simulink model "Model_2Systems"  (R2018b)
settings: Solver=ode23tb  StartTime=0.0  StopTime=20  RelTol=1e-3
values from neighbouring files (symbols this model uses):
  Ts = 0.01; Simulation.Ts = Ts    [Parameters.m]
undefined symbols (not defined in the file or in its folder): DiscIntNeverNeededParam, Kv, p01, p02, q01, q02, Simulation, Vr0
libraries: simulink x6
settings Model: Creator=oscar  LastModifiedBy=oscar
settings SolverCC: ZeroCrossAlgorithm=Adaptive
settings DataIOCC: OutputOption=SpecifiedOutputTimes  OutputTimes=t_out
settings SFSimCC: SimUseLocalCustomCode=off
settings RTWCC: RTWUseLocalCustomCode=off

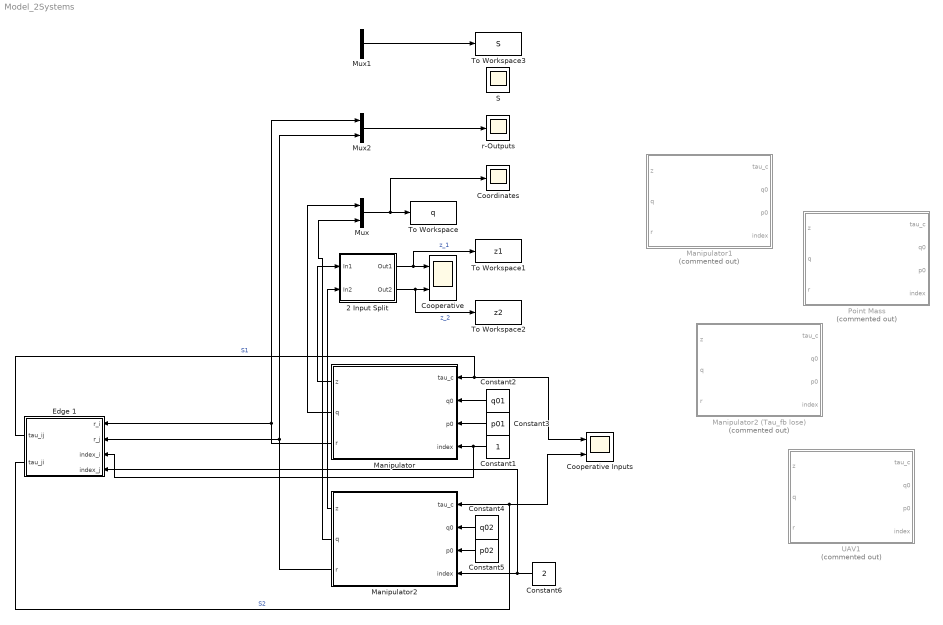
== system Model_2Systems ==
  2 Input Split : Subsystem
  Constant1 : Constant
  Constant2 : Constant  Value=q01
  Constant3 : Constant  Value=p01
  Constant4 : Constant  Value=q02
  Constant5 : Constant  Value=p02
  Constant6 : Constant  Value=2
  Cooperative : Scope  NumInputPorts=2
  Cooperative Inputs : Scope  NumInputPorts=2
  Coordinates : Scope
  Edge 1 : Subsystem
  Manipulator : Subsystem
  Manipulator1 : Subsystem  Commented=on
  Manipulator2 : Subsystem
  Manipulator2 (Tau_fb lose) : Subsystem  Commented=on
  Mux : Mux  Inputs=2
  Mux1 : Mux  Inputs=2
  Mux2 : Mux  Inputs=2
  Point Mass : Subsystem  Commented=on
  S : Scope  NumInputPorts=2
  To Workspace : ToWorkspace  VariableName=q  SaveFormat=Timeseries  SampleTime=-1
  To Workspace1 : ToWorkspace  VariableName=z1  SaveFormat=Timeseries  SampleTime=-1
  To Workspace2 : ToWorkspace  VariableName=z2  SaveFormat=Timeseries  SampleTime=-1
  To Workspace3 : ToWorkspace  VariableName=S  SaveFormat=Timeseries  SampleTime=-1
  UAV1 : Subsystem  Commented=on
  r-Outputs : Scope
  wires:
  Mux/1 -> Coordinates/1, To Workspace/1
  Manipulator/2(q) -> Mux/1
  Manipulator2/2(q) -> Mux/2
  Constant2/1 -> Manipulator/2(q0)
  Constant3/1 -> Manipulator/3(p0)
  Constant4/1 -> Manipulator2/2(q0)
  Constant5/1 -> Manipulator2/3(p0)
  Edge 1/1(tau_ij) -> Manipulator/1(tau_c), Cooperative Inputs/1  "S1"
  Edge 1/2(tau_ji) -> Manipulator2/1(tau_c), Cooperative Inputs/2  "S2"
  Manipulator2/3(r) -> Edge 1/2(r_j), Mux2/2
  Constant1/1 -> Manipulator/4(index), Edge 1/3(index_i)
  Constant6/1 -> Manipulator2/4(index), Edge 1/4(index_j)
  Manipulator/3(r) -> Edge 1/1(r_i), Mux2/1
  Mux2/1 -> r-Outputs/1
  Manipulator/1(z) -> 2 Input Split/1(In1)
  Manipulator2/1(z) -> 2 Input Split/2(In2)
  2 Input Split/1(Out1) -> To Workspace1/1, Cooperative/1  "z_1"
  2 Input Split/2(Out2) -> To Workspace2/1, Cooperative/2  "z_2"
  Mux1/1 -> To Workspace3/1

== system Model_2Systems/2 Input Split ==
  In1 : Inport
  In2 : Inport  Port=2
  Demux : Demux  Outputs=2
  Demux1 : Demux  Outputs=2
  Mux1 : Mux  Inputs=2
  Mux3 : Mux  Inputs=2
  Out1 : Outport
  Out2 : Outport  Port=2
  wires:
  Demux/1 -> Mux1/1
  Mux1/1 -> Out1/1
  In1/1 -> Demux/1
  Demux1/2 -> Mux3/2
  Mux3/1 -> Out2/1
  Demux1/1 -> Mux1/2
  Demux/2 -> Mux3/1
  In2/1 -> Demux1/1

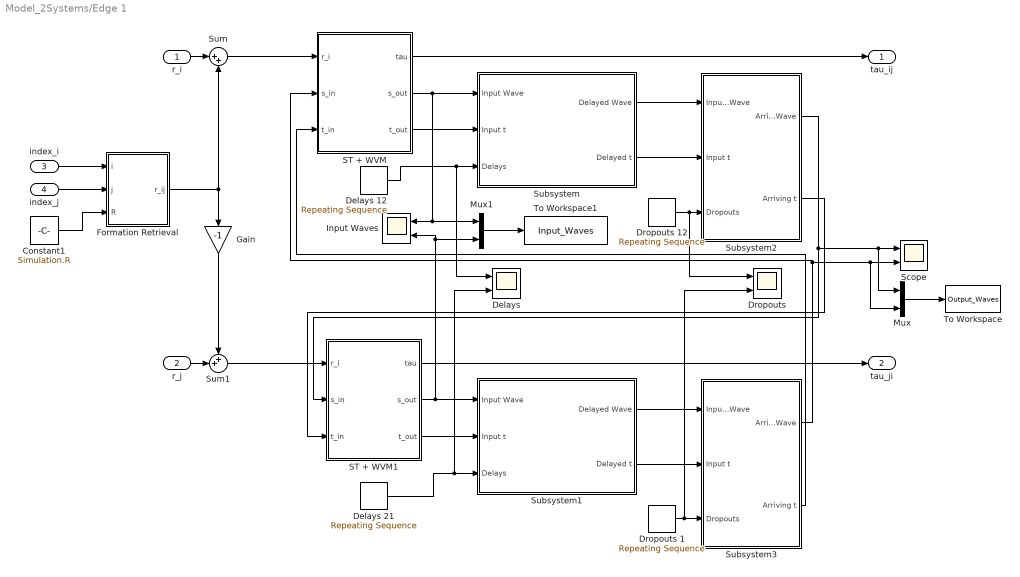
== system Model_2Systems/Edge 1 ==
  r_i : Inport
  r_j : Inport  Port=2
  index_i : Inport  Port=3
  index_j : Inport  Port=4
  Constant1 : Constant  Value=Simulation.R
  Delays : Scope  NumInputPorts=2
  Delays 12 : simulink/Sources/Repeating Sequence  rep_seq_t=t_delays  rep_seq_y=delays_12
  Delays 21 : simulink/Sources/Repeating Sequence  rep_seq_t=t_delays  rep_seq_y=delays_21
  Dropouts : Scope  NumInputPorts=2
  Dropouts 1 : simulink/Sources/Repeating Sequence  rep_seq_t=t_delays  rep_seq_y=dropouts_21
  Dropouts 12 : simulink/Sources/Repeating Sequence  rep_seq_t=t_delays  rep_seq_y=dropouts_12
  Formation Retrieval : MATLAB Function  TreatAsAtomicUnit=on
  Gain : Gain  Gain=-1
  Input Waves : Scope  NumInputPorts=2
  Mux : Mux  Inputs=2
  Mux1 : Mux  Inputs=2
  ST + WVM : Subsystem  TreatAsAtomicUnit=on
  ST + WVM1 : Subsystem  TreatAsAtomicUnit=on
  Scope : Scope  NumInputPorts=2
  Subsystem : Subsystem
  Subsystem1 : Subsystem
  Subsystem2 : Subsystem
  Subsystem3 : Subsystem
  Sum : Sum  Inputs=|++
  Sum1 : Sum  Inputs=++|
  To Workspace : ToWorkspace  VariableName=Output_Waves  SaveFormat=Timeseries  SampleTime=Ts
  To Workspace1 : ToWorkspace  VariableName=Input_Waves  SaveFormat=Timeseries  SampleTime=Ts
  tau_ij : Outport
  tau_ji : Outport  Port=2
  wires:
  r_i/1 -> Sum/1
  r_j/1 -> Sum1/2
  ST + WVM/1(tau) -> tau_ij/1
  Sum/1 -> ST + WVM/1(r_i)
  Sum1/1 -> ST + WVM1/1(r_i)
  index_i/1 -> Formation Retrieval/1(i)
  index_j/1 -> Formation Retrieval/2(j)
  Formation Retrieval/1(r_ij) -> Gain/1, Sum/2
  Gain/1 -> Sum1/1
  Constant1/1 -> Formation Retrieval/3(R)
  Delays 21/1 -> Delays/2, Subsystem1/3(Delays)
  ST + WVM/3(t_out) -> Subsystem/2(Input t)
  Delays 12/1 -> Delays/1, Subsystem/3(Delays)
  ST + WVM1/2(s_out) -> Subsystem1/1(Input Wave), Mux1/2, Input Waves/2
  ST + WVM1/3(t_out) -> Subsystem1/2(Input t)
  Subsystem/1(Delayed Wave) -> Subsystem2/1(Input Wave)
  ST + WVM1/1(tau) -> tau_ji/1
  Subsystem/2(Delayed t) -> Subsystem2/2(Input t)
  Dropouts 12/1 -> Dropouts/1, Subsystem2/3(Dropouts)
  Subsystem1/1(Delayed Wave) -> Subsystem3/1(Input Wave)
  Subsystem1/2(Delayed t) -> Subsystem3/2(Input t)
  Subsystem3/1(Arriving Wave) -> Mux/2, Scope/2, ST + WVM/2(s_in)
  Subsystem3/2(Arriving t) -> ST + WVM/3(t_in)
  Subsystem2/2(Arriving t) -> ST + WVM1/3(t_in)
  Subsystem2/1(Arriving Wave) -> ST + WVM1/2(s_in), Mux/1, Scope/1
  Dropouts 1/1 -> Subsystem3/3(Dropouts), Dropouts/2
  Mux/1 -> To Workspace/1
  ST + WVM/2(s_out) -> Subsystem/1(Input Wave), Input Waves/1, Mux1/1
  Mux1/1 -> To Workspace1/1

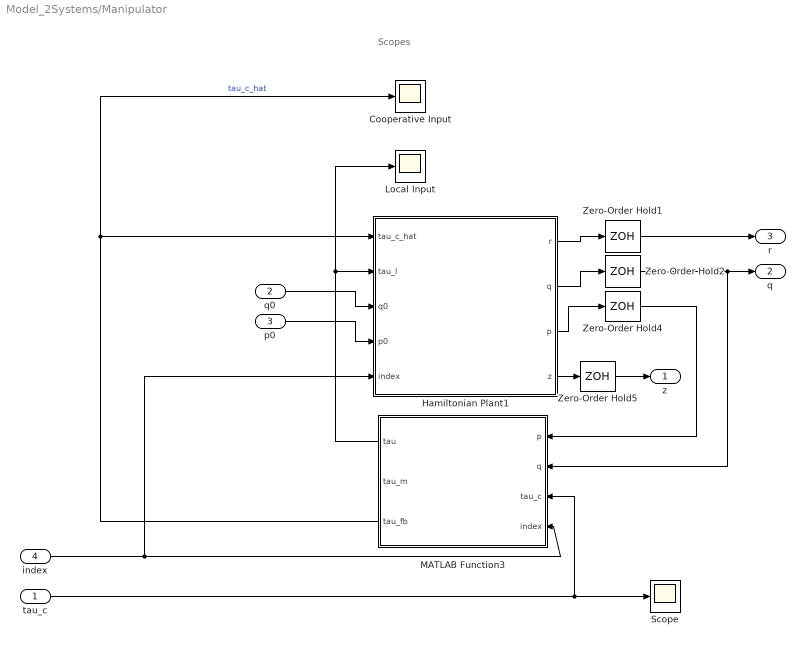
== system Model_2Systems/Manipulator ==
  note: Scopes
  tau_c : Inport
  q0 : Inport  Port=2
  p0 : Inport  Port=3
  index : Inport  Port=4
  Cooperative Input : Scope
  Hamiltonian Plant1 : Subsystem
  Local Input : Scope
  MATLAB Function3 : MATLAB Function  TreatAsAtomicUnit=on
  Scope : Scope
  Zero-Order Hold{1..2,4..5} (4 alike) : ZeroOrderHold  SampleTime=Ts
  z : Outport
  q : Outport  Port=2
  r : Outport  Port=3
  wires:
  Hamiltonian Plant1/2(q) -> Zero-Order Hold2/1
  index/1 -> Hamiltonian Plant1/5(index), MATLAB Function3/4(index)
  Hamiltonian Plant1/1(r) -> Zero-Order Hold1/1
  MATLAB Function3/1(tau) -> Local Input/1, Hamiltonian Plant1/2(tau_l)
  Hamiltonian Plant1/4(z) -> Zero-Order Hold5/1
  p0/1 -> Hamiltonian Plant1/4(p0)
  MATLAB Function3/3(tau_fb) -> Cooperative Input/1, Hamiltonian Plant1/1(tau_c_hat)  "tau_c_hat"
  Hamiltonian Plant1/3(p) -> Zero-Order Hold4/1
  q0/1 -> Hamiltonian Plant1/3(q0)
  Zero-Order Hold2/1 -> MATLAB Function3/2(q), q/1
  Zero-Order Hold4/1 -> MATLAB Function3/1(p)
  Zero-Order Hold1/1 -> r/1
  tau_c/1 -> Scope/1, MATLAB Function3/3(tau_c)
  Zero-Order Hold5/1 -> z/1

== system Model_2Systems/Manipulator1 ==
  tau_c : Inport
  q0 : Inport  Port=2
  p0 : Inport  Port=3
  index : Inport  Port=4
  Hamiltonian Plant : Subsystem
  Input Compensation : Scope  NumInputPorts=2
  Levenberg Compensation : MATLAB Function  Commented=on  TreatAsAtomicUnit=on
  Local Input : Scope
  MATLAB Function1 : MATLAB Function  TreatAsAtomicUnit=on
  Passivating Feedback : Scope
  Sum : Sum  Inputs=|++
  z : Outport
  q : Outport  Port=2
  r : Outport  Port=3
  wires:
  MATLAB Function1/1(tau) -> Hamiltonian Plant/3(tau_l), Local Input/1
  Hamiltonian Plant/4(p) -> MATLAB Function1/1(p)
  Hamiltonian Plant/3(q) -> q/1, MATLAB Function1/2(q)
  Hamiltonian Plant/5(z) -> z/1
  Hamiltonian Plant/2(r) -> r/1
  q0/1 -> Hamiltonian Plant/4(q0)
  p0/1 -> Hamiltonian Plant/5(p0)
  MATLAB Function1/2(tau_fb) -> Sum/2, Passivating Feedback/1
  index/1 -> Hamiltonian Plant/6(index), MATLAB Function1/3(index)
  Sum/1 -> Hamiltonian Plant/2(tau_c_hat), Input Compensation/2, Input Compensation/1  "tau_k"
  tau_c/1 -> Sum/1, Hamiltonian Plant/7(tau_c)  "tau_c_hat"

== system Model_2Systems/Manipulator2 ==
  note: Scopes
  tau_c : Inport
  q0 : Inport  Port=2
  p0 : Inport  Port=3
  index : Inport  Port=4
  Cooperative Input : Scope
  Hamiltonian Plant1 : Subsystem
  Local Input : Scope
  MATLAB Function3 : MATLAB Function  TreatAsAtomicUnit=on
  Scope : Scope
  Zero-Order Hold{1..2,4..5} (4 alike) : ZeroOrderHold  SampleTime=Ts
  z : Outport
  q : Outport  Port=2
  r : Outport  Port=3
  wires:
  Hamiltonian Plant1/2(q) -> Zero-Order Hold2/1
  index/1 -> Hamiltonian Plant1/5(index), MATLAB Function3/4(index)
  Hamiltonian Plant1/1(r) -> Zero-Order Hold1/1
  MATLAB Function3/1(tau) -> Local Input/1, Hamiltonian Plant1/2(tau_l)
  Hamiltonian Plant1/4(z) -> Zero-Order Hold5/1
  p0/1 -> Hamiltonian Plant1/4(p0)
  MATLAB Function3/3(tau_fb) -> Cooperative Input/1, Hamiltonian Plant1/1(tau_c_hat)  "tau_c_hat"
  Hamiltonian Plant1/3(p) -> Zero-Order Hold4/1
  q0/1 -> Hamiltonian Plant1/3(q0)
  Zero-Order Hold2/1 -> MATLAB Function3/2(q), q/1
  Zero-Order Hold4/1 -> MATLAB Function3/1(p)
  Zero-Order Hold1/1 -> r/1
  tau_c/1 -> Scope/1, MATLAB Function3/3(tau_c)
  Zero-Order Hold5/1 -> z/1

== system Model_2Systems/Manipulator2 (Tau_fb lose) ==
  tau_c : Inport
  q0 : Inport  Port=2
  p0 : Inport  Port=3
  index : Inport  Port=4
  Hamiltonian Plant : Subsystem
  Levenberg Compensation : MATLAB Function  Commented=on  TreatAsAtomicUnit=on
  Local Input : Scope
  MATLAB Function1 : MATLAB Function  TreatAsAtomicUnit=on
  MATLAB Function2 : MATLAB Function  Commented=on  TreatAsAtomicUnit=on
  Passivating Feedback : Scope
  Scope : Scope  NumInputPorts=4
  Sum : Sum  Inputs=|++
  System Input : Scope
  z : Outport
  q : Outport  Port=2
  r : Outport  Port=3
  wires:
  MATLAB Function1/1(tau) -> Hamiltonian Plant/2(tau_l), Local Input/1
  Hamiltonian Plant/3(p) -> MATLAB Function1/1(p)
  Hamiltonian Plant/2(q) -> MATLAB Function1/2(q), q/1
  Hamiltonian Plant/4(z) -> z/1
  Hamiltonian Plant/1(r) -> r/1
  q0/1 -> Hamiltonian Plant/3(q0)
  p0/1 -> Hamiltonian Plant/4(p0)
  MATLAB Function1/5(tau_fb) -> Scope/4, Sum/2, Passivating Feedback/1
  index/1 -> MATLAB Function1/3(index), Hamiltonian Plant/5(index)
  Sum/1 -> Hamiltonian Plant/1(tau_c_hat), System Input/1  "tau_k"
  tau_c/1 -> Sum/1, Hamiltonian Plant/6(tau_c)  "tau_c_hat"
  MATLAB Function1/2(tau_dH) -> Scope/1
  MATLAB Function1/3(tau_null) -> Scope/2
  MATLAB Function1/4(tau_lambda) -> Scope/3

== system Model_2Systems/Point Mass ==
  tau_c : Inport
  q0 : Inport  Port=2
  p0 : Inport  Port=3
  index : Inport  Port=4
  Hamiltonian Plant : Subsystem
  MATLAB Function1 : MATLAB Function  TreatAsAtomicUnit=on
  Scope : Scope
  Sum : Sum  Inputs=|++
  z : Outport
  q : Outport  Port=2
  r : Outport  Port=3
  wires:
  MATLAB Function1/1(tau) -> Hamiltonian Plant/2(tau_l)
  tau_c/1 -> Sum/1
  Hamiltonian Plant/3(p) -> MATLAB Function1/1(p)
  Hamiltonian Plant/2(q) -> MATLAB Function1/2(q), q/1
  Hamiltonian Plant/4(z) -> z/1
  Hamiltonian Plant/1(r) -> r/1
  q0/1 -> Hamiltonian Plant/3(q0)
  p0/1 -> Hamiltonian Plant/4(p0)
  MATLAB Function1/2(tau_fb) -> Scope/1, Sum/2
  Sum/1 -> Hamiltonian Plant/1(tau_c)
  index/1 -> Hamiltonian Plant/5(index), MATLAB Function1/3(index)

== system Model_2Systems/UAV1 ==
  tau_c : Inport
  q0 : Inport  Port=2
  p0 : Inport  Port=3
  index : Inport  Port=4
  Hamiltonian Plant : Subsystem
  Levenberg Compensation : MATLAB Function  Commented=on  TreatAsAtomicUnit=on
  Local Input : Scope
  MATLAB Function1 : MATLAB Function  TreatAsAtomicUnit=on
  Passivating Feedback : Scope
  Sum : Sum  Inputs=|++
  System Input : Scope
  z : Outport
  q : Outport  Port=2
  r : Outport  Port=3
  wires:
  MATLAB Function1/1(tau) -> Hamiltonian Plant/2(tau_l), Local Input/1
  Hamiltonian Plant/2(q) -> MATLAB Function1/2(q), q/1
  Hamiltonian Plant/4(z) -> z/1
  Hamiltonian Plant/1(r) -> r/1
  q0/1 -> Hamiltonian Plant/3(q0)
  p0/1 -> Hamiltonian Plant/4(p0)
  MATLAB Function1/2(tau_fb) -> Sum/2, Passivating Feedback/1
  index/1 -> MATLAB Function1/3(index), Hamiltonian Plant/5(index)
  Sum/1 -> System Input/1, Hamiltonian Plant/1(tau_c_hat)  "tau_c_hat"
  tau_c/1 -> Hamiltonian Plant/6(tau_c), Sum/1
  Hamiltonian Plant/3(p) -> MATLAB Function1/1(p)

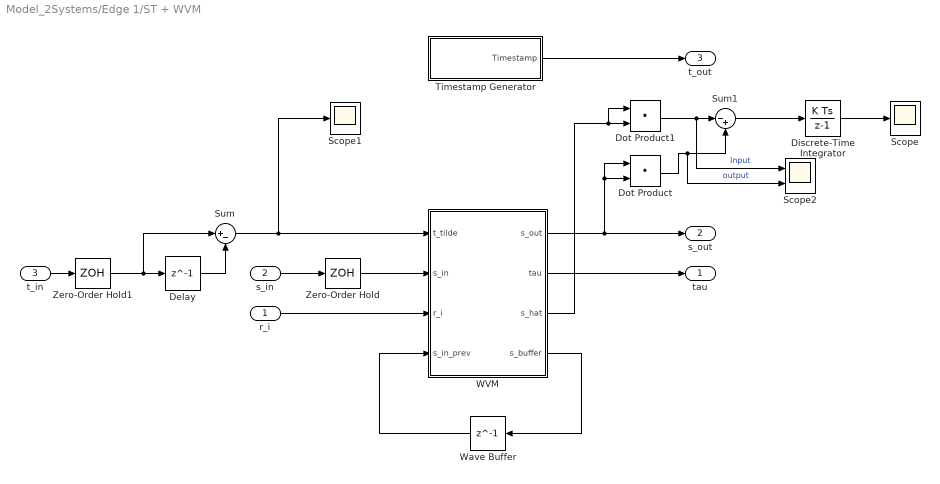
== system Model_2Systems/Edge 1/ST + WVM ==
  r_i : Inport
  s_in : Inport  Port=2
  t_in : Inport  Port=3
  Delay : Delay  DelayLength=1  SampleTime=Ts
  Discrete-Time Integrator : DiscreteIntegrator  SampleTime=-1  ICPrevOutput=DiscIntNeverNeededParam  ICPrevScaledInput=DiscIntNeverNeededParam
  Dot Product : DotProduct  InputSameDT=on  OutDataTypeStr=Inherit: Inherit via internal rule
  Dot Product1 : DotProduct  InputSameDT=on  OutDataTypeStr=Inherit: Inherit via internal rule
  Scope : Scope
  Scope1 : Scope
  Scope2 : Scope  NumInputPorts=2
  Sum : Sum  Inputs=|+-
  Sum1 : Sum  Inputs=|-+
  Timestamp Generator : Subsystem
  WVM : MATLAB Function  TreatAsAtomicUnit=on
  Wave Buffer : Delay  DelayLength=1  InitialCondition=[0;0]  SampleTime=Ts
  Zero-Order Hold : ZeroOrderHold  SampleTime=Ts
  Zero-Order Hold1 : ZeroOrderHold  SampleTime=Ts
  tau : Outport
  s_out : Outport  Port=2
  t_out : Outport  Port=3
  wires:
  t_in/1 -> Zero-Order Hold1/1
  Delay/1 -> Sum/2
  WVM/2(tau) -> tau/1
  WVM/1(s_out) -> Dot Product/2, Dot Product/1, s_out/1
  WVM/4(s_buffer) -> Wave Buffer/1
  Wave Buffer/1 -> WVM/4(s_in_prev)
  Sum/1 -> WVM/1(t_tilde), Scope1/1
  s_in/1 -> Zero-Order Hold/1
  r_i/1 -> WVM/3(r_i)
  WVM/3(s_hat) -> Dot Product1/1, Dot Product1/2
  Dot Product1/1 -> Scope2/1, Sum1/1  "Input"
  Dot Product/1 -> Scope2/2, Sum1/2  "output"
  Timestamp Generator/1(Timestamp) -> t_out/1
  Zero-Order Hold/1 -> WVM/2(s_in)
  Zero-Order Hold1/1 -> Sum/1, Delay/1
  Sum1/1 -> Discrete-Time Integrator/1
  Discrete-Time Integrator/1 -> Scope/1

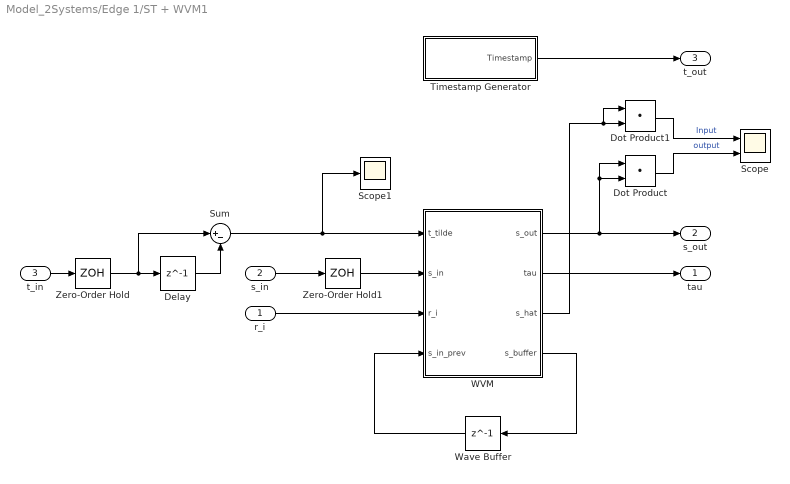
== system Model_2Systems/Edge 1/ST + WVM1 ==
  r_i : Inport
  s_in : Inport  Port=2
  t_in : Inport  Port=3
  Delay : Delay  DelayLength=1  SampleTime=Ts
  Dot Product : DotProduct  InputSameDT=on  OutDataTypeStr=Inherit: Inherit via internal rule
  Dot Product1 : DotProduct  InputSameDT=on  OutDataTypeStr=Inherit: Inherit via internal rule
  Scope : Scope  NumInputPorts=2
  Scope1 : Scope
  Sum : Sum  Inputs=|+-
  Timestamp Generator : Subsystem
  WVM : MATLAB Function  TreatAsAtomicUnit=on
  Wave Buffer : Delay  DelayLength=1  InitialCondition=[0;0]  SampleTime=Ts
  Zero-Order Hold : ZeroOrderHold  SampleTime=Ts
  Zero-Order Hold1 : ZeroOrderHold  SampleTime=Ts
  tau : Outport
  s_out : Outport  Port=2
  t_out : Outport  Port=3
  wires:
  t_in/1 -> Zero-Order Hold/1
  Delay/1 -> Sum/2
  WVM/2(tau) -> tau/1
  WVM/1(s_out) -> Dot Product/2, Dot Product/1, s_out/1
  WVM/4(s_buffer) -> Wave Buffer/1
  Wave Buffer/1 -> WVM/4(s_in_prev)
  Sum/1 -> Scope1/1, WVM/1(t_tilde)
  s_in/1 -> Zero-Order Hold1/1
  r_i/1 -> WVM/3(r_i)
  WVM/3(s_hat) -> Dot Product1/1, Dot Product1/2
  Dot Product1/1 -> Scope/1  "Input"
  Dot Product/1 -> Scope/2  "output"
  Timestamp Generator/1(Timestamp) -> t_out/1
  Zero-Order Hold1/1 -> WVM/2(s_in)
  Zero-Order Hold/1 -> Sum/1, Delay/1

== system Model_2Systems/Edge 1/Subsystem ==
  Input Wave : Inport
  Input t : Inport  Port=2
  Delays : Inport  Port=3
  Variable Integer Delay1 : Delay  DelayLengthSource=Input port  PreventDirectFeedthrough=on  SampleTime=Ts
      settings: InputPortMap=u0,p1
  Variable Integer Delay2 : Delay  DelayLengthSource=Input port  PreventDirectFeedthrough=on  SampleTime=Ts
      settings: InputPortMap=u0,p1
  Zero-Order Hold : ZeroOrderHold  SampleTime=Ts
  Delayed Wave : Outport
  Delayed t : Outport  Port=2
  wires:
  Input Wave/1 -> Variable Integer Delay2/1
  Input t/1 -> Variable Integer Delay1/1
  Variable Integer Delay2/1 -> Delayed Wave/1
  Variable Integer Delay1/1 -> Delayed t/1
  Delays/1 -> Zero-Order Hold/1
  Zero-Order Hold/1 -> Variable Integer Delay2/2, Variable Integer Delay1/2

== system Model_2Systems/Edge 1/Subsystem1 ==
  Input Wave : Inport
  Input t : Inport  Port=2
  Delays : Inport  Port=3
  Variable Integer Delay1 : Delay  DelayLengthSource=Input port  PreventDirectFeedthrough=on  SampleTime=Ts
      settings: InputPortMap=u0,p1
  Variable Integer Delay2 : Delay  DelayLengthSource=Input port  PreventDirectFeedthrough=on  SampleTime=Ts
      settings: InputPortMap=u0,p1
  Zero-Order Hold : ZeroOrderHold  SampleTime=Ts
  Delayed Wave : Outport
  Delayed t : Outport  Port=2
  wires:
  Input Wave/1 -> Variable Integer Delay2/1
  Zero-Order Hold/1 -> Variable Integer Delay2/2, Variable Integer Delay1/2
  Input t/1 -> Variable Integer Delay1/1
  Variable Integer Delay2/1 -> Delayed Wave/1
  Variable Integer Delay1/1 -> Delayed t/1
  Delays/1 -> Zero-Order Hold/1

== system Model_2Systems/Edge 1/Subsystem2 ==
  Input Wave : Inport
  Input t : Inport  Port=2
  Dropouts : Inport  Port=3
  Ground : Ground
  Ground1 : Ground
  Switch : Switch  Criteria=u2 > Threshold
  Switch1 : Switch  Criteria=u2 > Threshold
  Zero-Order Hold : ZeroOrderHold  SampleTime=Ts
  Arriving Wave : Outport
  Arriving t : Outport  Port=2
  wires:
  Input Wave/1 -> Switch/3
  Switch/1 -> Arriving Wave/1
  Switch1/1 -> Arriving t/1
  Dropouts/1 -> Zero-Order Hold/1
  Zero-Order Hold/1 -> Switch1/2, Switch/2
  Input t/1 -> Switch1/3
  Ground1/1 -> Switch/1
  Ground/1 -> Switch1/1

== system Model_2Systems/Edge 1/Subsystem3 ==
  Input Wave : Inport
  Input t : Inport  Port=2
  Dropouts : Inport  Port=3
  Ground1 : Ground
  Ground2 : Ground
  Switch : Switch  Criteria=u2 > Threshold
  Switch1 : Switch  Criteria=u2 > Threshold
  Zero-Order Hold : ZeroOrderHold  SampleTime=Ts
  Arriving Wave : Outport
  Arriving t : Outport  Port=2
  wires:
  Input Wave/1 -> Switch/3
  Switch/1 -> Arriving Wave/1
  Switch1/1 -> Arriving t/1
  Dropouts/1 -> Zero-Order Hold/1
  Zero-Order Hold/1 -> Switch1/2, Switch/2
  Input t/1 -> Switch1/3
  Ground1/1 -> Switch/1
  Ground2/1 -> Switch1/1

== system Model_2Systems/Manipulator/Hamiltonian Plant1 ==
  tau_c_hat : Inport
  tau_l : Inport  Port=2
  q0 : Inport  Port=3
  p0 : Inport  Port=4
  index : Inport  Port=5
  Integrator : Integrator  InitialConditionSource=external  InitialCondition=q01
  Integrator1 : Integrator  InitialConditionSource=external  InitialCondition=p02
  MATLAB Function1 : MATLAB Function  TreatAsAtomicUnit=on
  MATLAB Function2 : MATLAB Function  TreatAsAtomicUnit=on
  r : Outport
  q : Outport  Port=2
  p : Outport  Port=3
  z : Outport  Port=4
  wires:
  tau_l/1 -> MATLAB Function2/3(tau_l)
  MATLAB Function2/2(pdot) -> Integrator1/1
  Integrator1/1 -> MATLAB Function2/2(p), p/1, MATLAB Function1/2(p)
  Integrator/1 -> q/1, MATLAB Function2/1(q), MATLAB Function1/1(q)
  MATLAB Function2/1(qdot) -> Integrator/1
  p0/1 -> Integrator1/2
  q0/1 -> Integrator/2
  MATLAB Function1/1(z_out) -> z/1
  MATLAB Function1/2(r_out) -> r/1
  index/1 -> MATLAB Function1/3(index), MATLAB Function2/5(index)
  tau_c_hat/1 -> MATLAB Function2/4(tau_c)

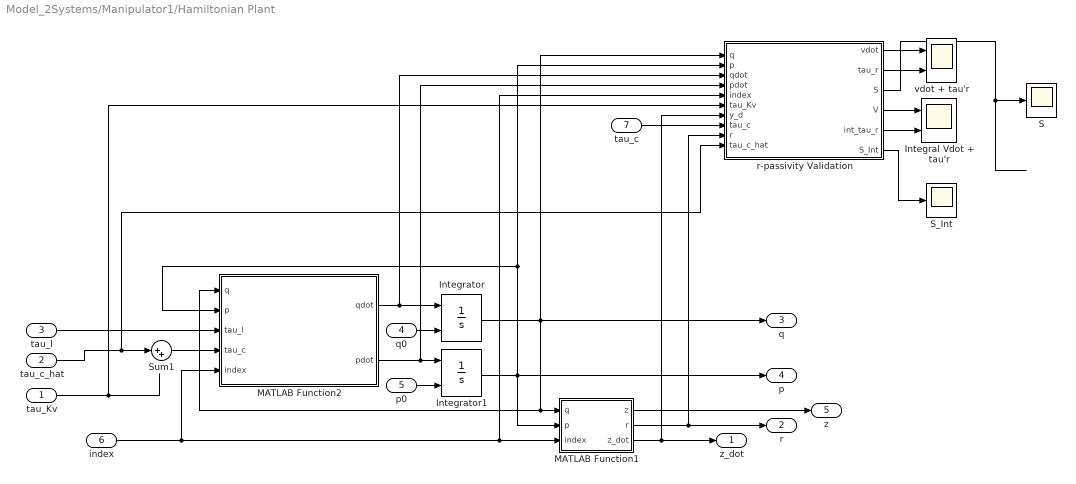
== system Model_2Systems/Manipulator1/Hamiltonian Plant ==
  tau_Kv : Inport
  tau_c_hat : Inport  Port=2
  tau_l : Inport  Port=3
  q0 : Inport  Port=4
  p0 : Inport  Port=5
  index : Inport  Port=6
  tau_c : Inport  Port=7
  Integral Vdot + tau'r : Scope  NumInputPorts=2
  Integrator : Integrator  InitialConditionSource=external  InitialCondition=q01
  Integrator1 : Integrator  InitialConditionSource=external  InitialCondition=p02
  MATLAB Function1 : MATLAB Function  TreatAsAtomicUnit=on
  MATLAB Function2 : MATLAB Function  TreatAsAtomicUnit=on
  S : Scope
  S_Int : Scope
  Sum1 : Sum  Inputs=|++
  r-passivity Validation : Subsystem
  vdot + tau'r : Scope  NumInputPorts=2
  z_dot : Outport
  r : Outport  Port=2
  q : Outport  Port=3
  p : Outport  Port=4
  z : Outport  Port=5
  wires:
  tau_l/1 -> MATLAB Function2/3(tau_l)
  MATLAB Function2/2(pdot) -> r-passivity Validation/4(pdot), Integrator1/1
  Integrator1/1 -> r-passivity Validation/2(p), MATLAB Function2/2(p), p/1, MATLAB Function1/2(p)
  Integrator/1 -> r-passivity Validation/1(q), q/1, MATLAB Function2/1(q), MATLAB Function1/1(q)
  MATLAB Function2/1(qdot) -> r-passivity Validation/3(qdot), Integrator/1
  p0/1 -> Integrator1/2
  tau_c_hat/1 -> r-passivity Validation/10(tau_c_hat), Sum1/1
  q0/1 -> Integrator/2
  MATLAB Function1/1(z) -> z/1
  MATLAB Function1/2(r) -> r-passivity Validation/9(r), r/1
  index/1 -> r-passivity Validation/5(index), MATLAB Function1/3(index), MATLAB Function2/5(index)
  MATLAB Function1/3(z_dot) -> r-passivity Validation/7(y_d), z_dot/1
  r-passivity Validation/1(vdot) -> vdot + tau'r/1
  r-passivity Validation/2(tau_r) -> vdot + tau'r/2
  r-passivity Validation/5(int_tau_r) -> Integral Vdot + tau'r/2
  r-passivity Validation/4(V) -> Integral Vdot + tau'r/1
  r-passivity Validation/3(S) -> S/1
  tau_c/1 -> r-passivity Validation/8(tau_c)
  tau_Kv/1 -> r-passivity Validation/6(tau_Kv)
  Sum1/1 -> MATLAB Function2/4(tau_c)
  r-passivity Validation/6(S_Int) -> S_Int/1

== system Model_2Systems/Manipulator2/Hamiltonian Plant1 ==
  tau_c_hat : Inport
  tau_l : Inport  Port=2
  q0 : Inport  Port=3
  p0 : Inport  Port=4
  index : Inport  Port=5
  Integrator : Integrator  InitialConditionSource=external  InitialCondition=q01
  Integrator1 : Integrator  InitialConditionSource=external  InitialCondition=p02
  MATLAB Function1 : MATLAB Function  TreatAsAtomicUnit=on
  MATLAB Function2 : MATLAB Function  TreatAsAtomicUnit=on
  r : Outport
  q : Outport  Port=2
  p : Outport  Port=3
  z : Outport  Port=4
  wires:
  tau_l/1 -> MATLAB Function2/3(tau_l)
  MATLAB Function2/2(pdot) -> Integrator1/1
  Integrator1/1 -> MATLAB Function2/2(p), p/1, MATLAB Function1/2(p)
  Integrator/1 -> q/1, MATLAB Function2/1(q), MATLAB Function1/1(q)
  MATLAB Function2/1(qdot) -> Integrator/1
  p0/1 -> Integrator1/2
  q0/1 -> Integrator/2
  MATLAB Function1/1(z_out) -> z/1
  MATLAB Function1/2(r_out) -> r/1
  index/1 -> MATLAB Function1/3(index), MATLAB Function2/5(index)
  tau_c_hat/1 -> MATLAB Function2/4(tau_c)

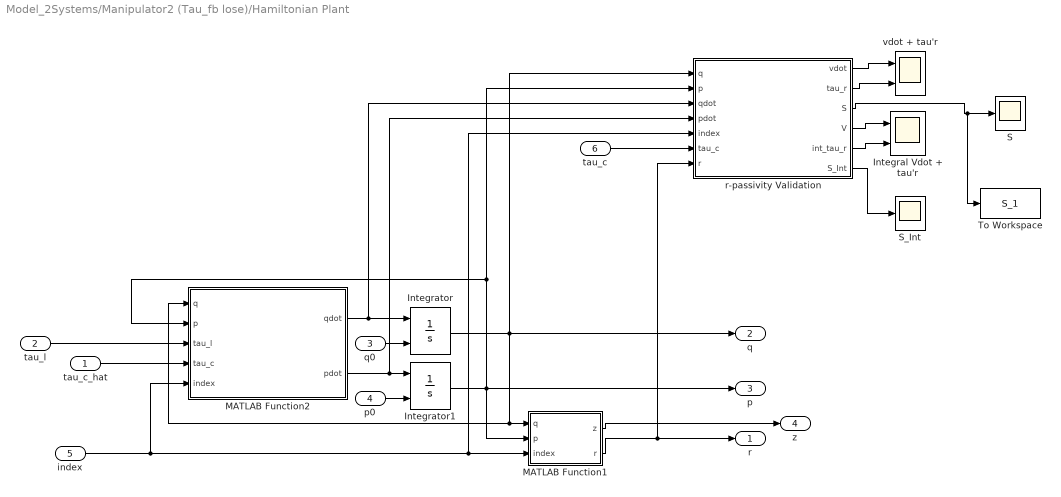
== system Model_2Systems/Manipulator2 (Tau_fb lose)/Hamiltonian Plant ==
  tau_c_hat : Inport
  tau_l : Inport  Port=2
  q0 : Inport  Port=3
  p0 : Inport  Port=4
  index : Inport  Port=5
  tau_c : Inport  Port=6
  Integral Vdot + tau'r : Scope  NumInputPorts=2
  Integrator : Integrator  InitialConditionSource=external  InitialCondition=q01
  Integrator1 : Integrator  InitialConditionSource=external  InitialCondition=p02
  MATLAB Function1 : MATLAB Function  TreatAsAtomicUnit=on
  MATLAB Function2 : MATLAB Function  TreatAsAtomicUnit=on
  S : Scope
  S_Int : Scope
  To Workspace : ToWorkspace  VariableName=S_1  SaveFormat=Timeseries  SampleTime=-1
  r-passivity Validation : Subsystem
  vdot + tau'r : Scope  NumInputPorts=2
  r : Outport
  q : Outport  Port=2
  p : Outport  Port=3
  z : Outport  Port=4
  wires:
  tau_l/1 -> MATLAB Function2/3(tau_l)
  MATLAB Function2/2(pdot) -> r-passivity Validation/4(pdot), Integrator1/1
  Integrator1/1 -> r-passivity Validation/2(p), MATLAB Function2/2(p), p/1, MATLAB Function1/2(p)
  Integrator/1 -> r-passivity Validation/1(q), q/1, MATLAB Function2/1(q), MATLAB Function1/1(q)
  MATLAB Function2/1(qdot) -> r-passivity Validation/3(qdot), Integrator/1
  p0/1 -> Integrator1/2
  q0/1 -> Integrator/2
  MATLAB Function1/1(z) -> z/1
  MATLAB Function1/2(r) -> r-passivity Validation/7(r), r/1
  index/1 -> r-passivity Validation/5(index), MATLAB Function1/3(index), MATLAB Function2/5(index)
  r-passivity Validation/1(vdot) -> vdot + tau'r/1
  r-passivity Validation/2(tau_r) -> vdot + tau'r/2
  r-passivity Validation/5(int_tau_r) -> Integral Vdot + tau'r/2
  r-passivity Validation/4(V) -> Integral Vdot + tau'r/1
  r-passivity Validation/3(S) -> To Workspace/1, S/1
  tau_c/1 -> r-passivity Validation/6(tau_c)
  tau_c_hat/1 -> MATLAB Function2/4(tau_c)
  r-passivity Validation/6(S_Int) -> S_Int/1

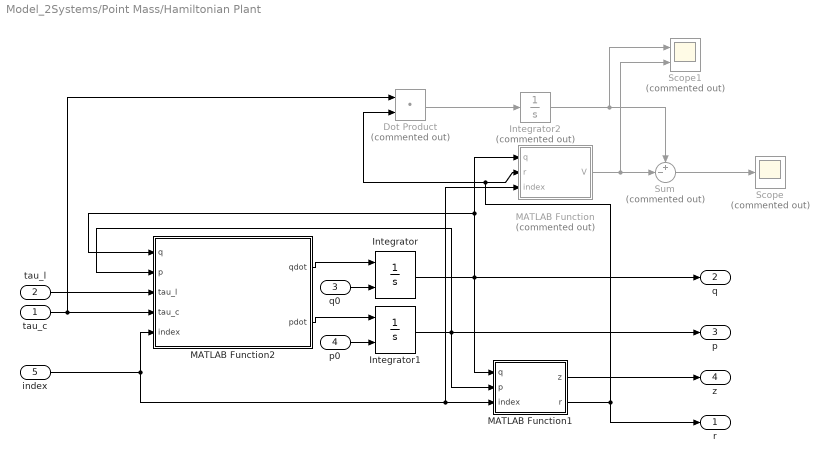
== system Model_2Systems/Point Mass/Hamiltonian Plant ==
  tau_c : Inport
  tau_l : Inport  Port=2
  q0 : Inport  Port=3
  p0 : Inport  Port=4
  index : Inport  Port=5
  Dot Product : DotProduct  Commented=on  InputSameDT=on  OutDataTypeStr=Inherit: Inherit via internal rule
  Integrator : Integrator  InitialConditionSource=external  InitialCondition=q01
  Integrator1 : Integrator  InitialConditionSource=external  InitialCondition=p02
  Integrator2 : Integrator  Commented=on
  MATLAB Function : MATLAB Function  Commented=on  TreatAsAtomicUnit=on
  MATLAB Function1 : MATLAB Function  TreatAsAtomicUnit=on
  MATLAB Function2 : MATLAB Function  TreatAsAtomicUnit=on
  Scope : Scope  Commented=on
  Scope1 : Scope  Commented=on  NumInputPorts=2
  Sum : Sum  Commented=on  Inputs=+-|
  r : Outport
  q : Outport  Port=2
  p : Outport  Port=3
  z : Outport  Port=4
  wires:
  tau_l/1 -> MATLAB Function2/3(tau_l)
  MATLAB Function2/2(pdot) -> Integrator1/1
  Integrator1/1 -> MATLAB Function1/2(p), MATLAB Function2/2(p), p/1
  Integrator/1 -> MATLAB Function1/1(q), MATLAB Function/1(q), MATLAB Function2/1(q), q/1
  MATLAB Function2/1(qdot) -> Integrator/1
  p0/1 -> Integrator1/2
  tau_c/1 -> MATLAB Function2/4(tau_c), Dot Product/1
  q0/1 -> Integrator/2
  MATLAB Function/1(V) -> Scope1/2, Sum/2
  Dot Product/1 -> Integrator2/1
  Sum/1 -> Scope/1
  Integrator2/1 -> Scope1/1, Sum/1
  MATLAB Function1/1(z) -> z/1
  MATLAB Function1/2(r) -> MATLAB Function/2(r), Dot Product/2, r/1
  index/1 -> MATLAB Function/3(index), MATLAB Function1/3(index), MATLAB Function2/5(index)

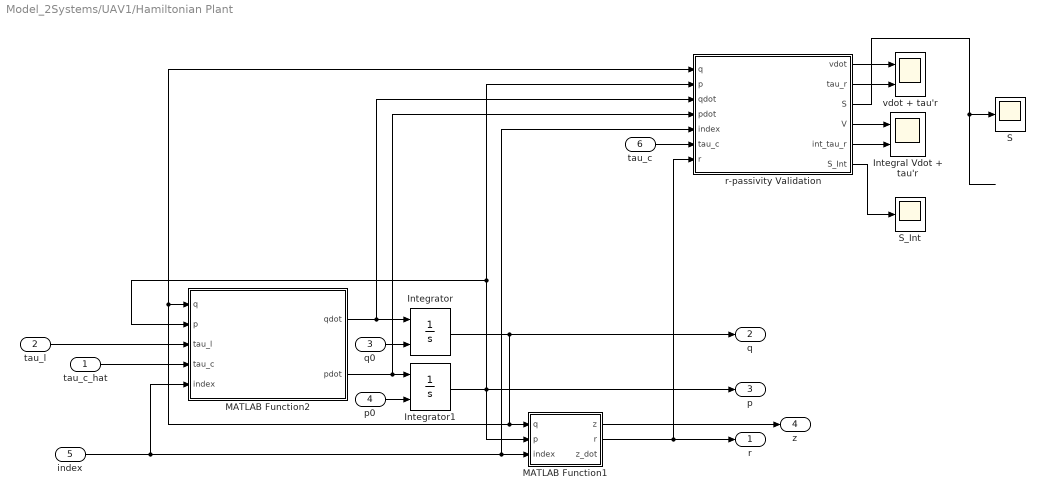
== system Model_2Systems/UAV1/Hamiltonian Plant ==
  tau_c_hat : Inport
  tau_l : Inport  Port=2
  q0 : Inport  Port=3
  p0 : Inport  Port=4
  index : Inport  Port=5
  tau_c : Inport  Port=6
  Integral Vdot + tau'r : Scope  NumInputPorts=2
  Integrator : Integrator  InitialConditionSource=external  InitialCondition=q01
  Integrator1 : Integrator  InitialConditionSource=external  InitialCondition=p02
  MATLAB Function1 : MATLAB Function  TreatAsAtomicUnit=on
  MATLAB Function2 : MATLAB Function  TreatAsAtomicUnit=on
  S : Scope
  S_Int : Scope
  r-passivity Validation : Subsystem
  vdot + tau'r : Scope  NumInputPorts=2
  r : Outport
  q : Outport  Port=2
  p : Outport  Port=3
  z : Outport  Port=4
  wires:
  tau_l/1 -> MATLAB Function2/3(tau_l)
  MATLAB Function2/2(pdot) -> r-passivity Validation/4(pdot), Integrator1/1
  Integrator1/1 -> MATLAB Function2/2(p), r-passivity Validation/2(p), p/1, MATLAB Function1/2(p)
  Integrator/1 -> q/1, r-passivity Validation/1(q), MATLAB Function2/1(q), MATLAB Function1/1(q)
  MATLAB Function2/1(qdot) -> r-passivity Validation/3(qdot), Integrator/1
  p0/1 -> Integrator1/2
  q0/1 -> Integrator/2
  MATLAB Function1/1(z) -> z/1
  MATLAB Function1/2(r) -> r-passivity Validation/7(r), r/1
  index/1 -> r-passivity Validation/5(index), MATLAB Function1/3(index), MATLAB Function2/5(index)
  r-passivity Validation/1(vdot) -> vdot + tau'r/1
  r-passivity Validation/2(tau_r) -> vdot + tau'r/2
  r-passivity Validation/5(int_tau_r) -> Integral Vdot + tau'r/2
  r-passivity Validation/4(V) -> Integral Vdot + tau'r/1
  r-passivity Validation/3(S) -> S/1
  tau_c_hat/1 -> MATLAB Function2/4(tau_c)
  r-passivity Validation/6(S_Int) -> S_Int/1
  tau_c/1 -> r-passivity Validation/6(tau_c)

== system Model_2Systems/Edge 1/ST + WVM/Timestamp Generator ==
  note: Timestamp
  Ramp1 : simulink/Sources/Ramp  slope=1/Ts  start=0  InitialOutput=0
  Rounding Function : Rounding
  Timestamp : Outport
  wires:
  Rounding Function/1 -> Timestamp/1
  Ramp1/1 -> Rounding Function/1

== system Model_2Systems/Edge 1/ST + WVM1/Timestamp Generator ==
  note: Timestamp
  Ramp1 : simulink/Sources/Ramp  slope=1/Ts  start=0  InitialOutput=0
  Rounding Function : Rounding
  Timestamp : Outport
  wires:
  Rounding Function/1 -> Timestamp/1
  Ramp1/1 -> Rounding Function/1

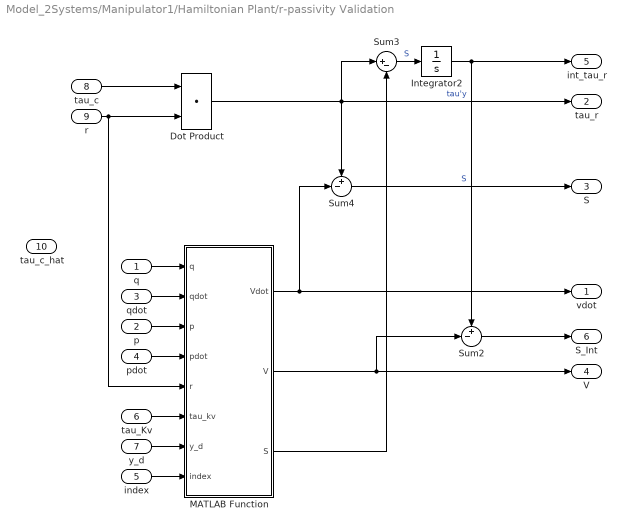
== system Model_2Systems/Manipulator1/Hamiltonian Plant/r-passivity Validation ==
  q : Inport
  p : Inport  Port=2
  qdot : Inport  Port=3
  pdot : Inport  Port=4
  index : Inport  Port=5
  tau_Kv : Inport  Port=6
  y_d : Inport  Port=7
  tau_c : Inport  Port=8
  r : Inport  Port=9
  tau_c_hat : Inport  Port=10
  Dot Product : DotProduct  InputSameDT=on  OutDataTypeStr=Inherit: Inherit via internal rule
  Integrator2 : Integrator
  MATLAB Function : MATLAB Function  TreatAsAtomicUnit=on
  Sum2 : Sum  Inputs=+-|
  Sum3 : Sum  Inputs=|+-
  Sum4 : Sum  Inputs=+-|
  vdot : Outport
  tau_r : Outport  Port=2
  S : Outport  Port=3
  V : Outport  Port=4
  int_tau_r : Outport  Port=5
  S_Int : Outport  Port=6
  wires:
  Sum4/1 -> S/1  "S"
  pdot/1 -> MATLAB Function/4(pdot)
  p/1 -> MATLAB Function/3(p)
  qdot/1 -> MATLAB Function/2(qdot)
  index/1 -> MATLAB Function/8(index)
  q/1 -> MATLAB Function/1(q)
  tau_Kv/1 -> MATLAB Function/6(tau_kv)
  y_d/1 -> MATLAB Function/7(y_d)
  tau_c/1 -> Dot Product/1
  r/1 -> Dot Product/2, MATLAB Function/5(r)
  Dot Product/1 -> Sum3/1, tau_r/1, Sum4/1  "tau'y"
  MATLAB Function/1(Vdot) -> Sum4/2, vdot/1
  MATLAB Function/2(V) -> Sum2/2, V/1
  Integrator2/1 -> int_tau_r/1, Sum2/1
  Sum2/1 -> S_Int/1
  MATLAB Function/3(S) -> Sum3/2
  Sum3/1 -> Integrator2/1  "S"

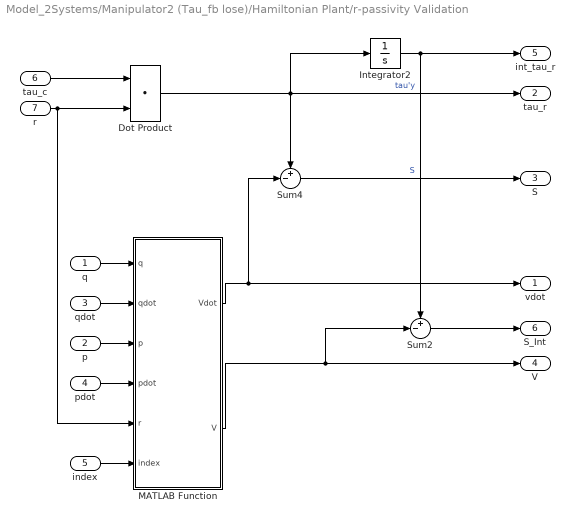
== system Model_2Systems/Manipulator2 (Tau_fb lose)/Hamiltonian Plant/r-passivity Validation ==
  q : Inport
  p : Inport  Port=2
  qdot : Inport  Port=3
  pdot : Inport  Port=4
  index : Inport  Port=5
  tau_c : Inport  Port=6
  r : Inport  Port=7
  Dot Product : DotProduct  InputSameDT=on  OutDataTypeStr=Inherit: Inherit via internal rule
  Integrator2 : Integrator
  MATLAB Function : MATLAB Function  TreatAsAtomicUnit=on
  Sum2 : Sum  Inputs=+-|
  Sum4 : Sum  Inputs=+-|
  vdot : Outport
  tau_r : Outport  Port=2
  S : Outport  Port=3
  V : Outport  Port=4
  int_tau_r : Outport  Port=5
  S_Int : Outport  Port=6
  wires:
  Sum4/1 -> S/1  "S"
  pdot/1 -> MATLAB Function/4(pdot)
  p/1 -> MATLAB Function/3(p)
  qdot/1 -> MATLAB Function/2(qdot)
  index/1 -> MATLAB Function/6(index)
  q/1 -> MATLAB Function/1(q)
  tau_c/1 -> Dot Product/1
  r/1 -> Dot Product/2, MATLAB Function/5(r)
  Dot Product/1 -> Integrator2/1, tau_r/1, Sum4/1  "tau'y"
  MATLAB Function/1(Vdot) -> Sum4/2, vdot/1
  MATLAB Function/2(V) -> Sum2/2, V/1
  Integrator2/1 -> int_tau_r/1, Sum2/1
  Sum2/1 -> S_Int/1

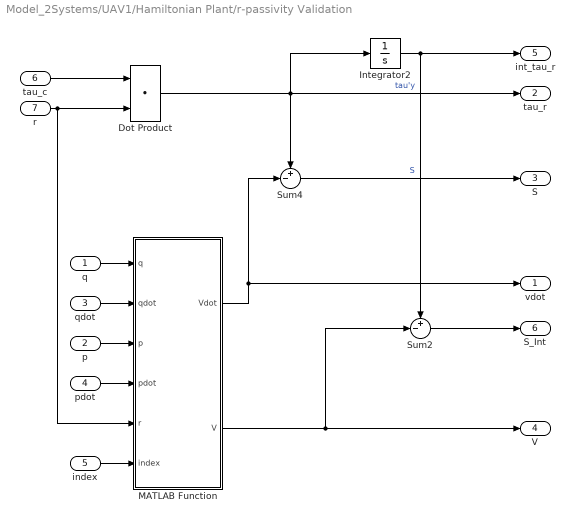
== system Model_2Systems/UAV1/Hamiltonian Plant/r-passivity Validation ==
  q : Inport
  p : Inport  Port=2
  qdot : Inport  Port=3
  pdot : Inport  Port=4
  index : Inport  Port=5
  tau_c : Inport  Port=6
  r : Inport  Port=7
  Dot Product : DotProduct  InputSameDT=on  OutDataTypeStr=Inherit: Inherit via internal rule
  Integrator2 : Integrator
  MATLAB Function : MATLAB Function  TreatAsAtomicUnit=on
  Sum2 : Sum  Inputs=+-|
  Sum4 : Sum  Inputs=+-|
  vdot : Outport
  tau_r : Outport  Port=2
  S : Outport  Port=3
  V : Outport  Port=4
  int_tau_r : Outport  Port=5
  S_Int : Outport  Port=6
  wires:
  Sum4/1 -> S/1  "S"
  pdot/1 -> MATLAB Function/4(pdot)
  p/1 -> MATLAB Function/3(p)
  qdot/1 -> MATLAB Function/2(qdot)
  index/1 -> MATLAB Function/6(index)
  q/1 -> MATLAB Function/1(q)
  tau_c/1 -> Dot Product/1
  r/1 -> Dot Product/2, MATLAB Function/5(r)
  Dot Product/1 -> Integrator2/1, tau_r/1, Sum4/1  "tau'y"
  MATLAB Function/1(Vdot) -> Sum4/2, vdot/1
  MATLAB Function/2(V) -> Sum2/2, V/1
  Integrator2/1 -> int_tau_r/1, Sum2/1
  Sum2/1 -> S_Int/1

== matlab function Model_2Systems/Point Mass/Hamiltonian Plant/MATLAB Function ==
  data: q input; r input; index input; V output; Vr0 parameter
function V = fcn(q, r, index, Vr0)

%     coder.extrinsic('R_Validation');
%     V = 0;
%     [V] = R_Validation(q, r, index);
%     V = V - Vr0;
V = 0;
end

== matlab function Model_2Systems/Point Mass/Hamiltonian Plant/MATLAB Function1 ==
  data: q input; z output; p input; r output; index input
function [z, r] = toz(q, p, index)

    coder.extrinsic('Pointmass2D_z');
    z = zeros(2, 1);
    r = zeros(2, 1);    
    [z, r] = Pointmass2D_z(q, p, index);

== matlab function Model_2Systems/UAV1/Hamiltonian Plant/MATLAB Function1 ==
  data: q input; z output; p input; r output; index input; z_dot output
function [z, r, z_dot] = toz(q, p, index)

    coder.extrinsic('UAV_z');
    z = zeros(2, 1);
    r = zeros(2, 1);
    z_dot = zeros(2, 1);
    [z, r, z_dot] = UAV_z(q, p, index);

== matlab function Model_2Systems/UAV1/Hamiltonian Plant/MATLAB Function2 ==
  data: q input; qdot output; p input; tau_l input; pdot output; tau_c input; index input
function [qdot, pdot] = fcn(q, p, tau_l, tau_c, index)

    coder.extrinsic('UAV_Dynamics');
    qdot = zeros(3, 1);
    pdot = zeros(3, 1);
    [qdot, pdot] = UAV_Dynamics(q, p, tau_l, tau_c, index);

== matlab function Model_2Systems/Point Mass/Hamiltonian Plant/MATLAB Function2 ==
  data: q input; qdot output; p input; tau_l input; pdot output; tau_c input; index input
function [qdot, pdot] = fcn(q, p, tau_l, tau_c, index)

    coder.extrinsic('Pointmass2D_Dynamics');
    qdot = zeros(2, 1);
    pdot = zeros(2, 1);
    [qdot, pdot] = Pointmass2D_Dynamics(q, p, tau_l, tau_c, index);

== matlab function Model_2Systems/Point Mass/MATLAB Function1 ==
  data: p input; q input; tau output; tau_fb output; index input
function [tau, tau_fb] = LocalControl(p, q, index)
    

coder.extrinsic('Pointmass2D_Control');
tau = zeros(2, 1);
tau_fb = zeros(2, 1);
[tau, tau_fb] = Pointmass2D_Control(q, p, index);

== matlab function Model_2Systems/Manipulator1/Hamiltonian Plant/MATLAB Function1 ==
  data: q input; z output; p input; r output; index input; z_dot output
function [z, r, z_dot] = toz(q, p, index)

    coder.extrinsic('Manipulator_z');
    z = zeros(2, 1);
    r = zeros(2, 1);
    z_dot = zeros(2, 1);
    [z, r, z_dot] = Manipulator_z(q, p, index);

== matlab function Model_2Systems/Manipulator1/Hamiltonian Plant/MATLAB Function2 ==
  data: q input; qdot output; p input; tau_l input; pdot output; tau_c input; index input
function [qdot, pdot] = fcn(q, p, tau_l, tau_c, index)

    coder.extrinsic('Manipulator_Dynamics');
    qdot = zeros(3, 1);
    pdot = zeros(3, 1);
    [qdot, pdot] = Manipulator_Dynamics(q, p, tau_l, tau_c, index);

== matlab function Model_2Systems/Manipulator1/Hamiltonian Plant/r-passivity Validation/MATLAB Function ==
  data: Vdot output; q input; qdot input; p input; pdot input; r input; tau_kv input; y_d input; index input; V output; Vr0 parameter; S output; Kv parameter
function [Vdot, V, S] = fcn(q, qdot, p, pdot, r, tau_kv, y_d, index, Vr0, Kv)

    coder.extrinsic('R_Validation');
    V = zeros(1,1); Vdot = 0; S = 0;
    [V, Vdot, S] = R_Validation(q, qdot,p, pdot, r, tau_kv, y_d, Kv, index);
    V = V - Vr0;
end

== matlab function Model_2Systems/Manipulator1/Levenberg Compensation ==
  data: q input; tau_k input; z_dot input; tau_c output; index input
function tau_c  = Pre(q, tau_k, z_dot, index)

    coder.extrinsic('Manipulator_Pre');
    tau_c = zeros(2,1);
    [tau_c] = Manipulator_Pre(q, tau_k, z_dot, index);
end

== matlab function Model_2Systems/Edge 1/Formation Retrieval ==
  data: i input; r_ij output; j input; R input
function r_ij = get_rij(i, j, R)
    %r_ij = zeros(2,1);
    r_ij = [R((i - 1)*2 + 1, j);R(2*i, j)];
end

== matlab function Model_2Systems/UAV1/Hamiltonian Plant/r-passivity Validation/MATLAB Function ==
  data: Vdot output; q input; qdot input; p input; pdot input; r input; index input; V output; Vr0 parameter
function [Vdot, V] = fcn(q, qdot, p, pdot, r, index, Vr0)

    coder.extrinsic('UAV_R');
    V = 0; Vdot = 0;
    [V, Vdot] = UAV_R(q, qdot,p, pdot, r, index);
    V = V - Vr0;
end

== matlab function Model_2Systems/UAV1/Levenberg Compensation ==
  data: q input; tau_k input; z_dot input; tau_c output; index input
function tau_c  = Pre(q, tau_k, z_dot, index)

    coder.extrinsic('Manipulator_Pre');
    tau_c = zeros(2,1);
    [tau_c] = Manipulator_Pre(q, tau_k, z_dot, index);
end

== matlab function Model_2Systems/UAV1/MATLAB Function1 ==
  data: p input; q input; tau output; tau_fb output; index input
function [tau, tau_fb] = LocalControl(p, q, index)
    

coder.extrinsic('UAV_Control');
tau = zeros(2, 1);
tau_fb = zeros(2, 1);
tau_Kv = zeros(2, 1);
[tau, tau_fb] = UAV_Control(q, p, index);

== matlab function Model_2Systems/Manipulator1/MATLAB Function1 ==
  data: p input; q input; tau output; tau_fb output; index input
function [tau, tau_fb] = LocalControl(p, q, index)
    

coder.extrinsic('Manipulator_Control');
tau = zeros(3, 1);
tau_fb = zeros(2, 1);
tau_Kv = zeros(2, 1);
[tau, tau_fb] = Manipulator_Control(q, p, index);

== matlab function Model_2Systems/Manipulator2 (Tau_fb lose)/Hamiltonian Plant/MATLAB Function1 ==
  data: q input; z output; p input; r output; index input
function [z, r] = toz(q, p, index)

    coder.extrinsic('Manipulator_z');
    z = zeros(2, 1);
    r = zeros(2, 1);
    [z, r] = Manipulator_z(q, p, index);

== matlab function Model_2Systems/Manipulator2 (Tau_fb lose)/Hamiltonian Plant/MATLAB Function2 ==
  data: q input; qdot output; p input; tau_l input; pdot output; tau_c input; index input
function [qdot, pdot] = fcn(q, p, tau_l, tau_c, index)

    coder.extrinsic('Manipulator_Dynamics');
    qdot = zeros(3, 1);
    pdot = zeros(3, 1);
    [qdot, pdot] = Manipulator_Dynamics(q, p, tau_l, tau_c, index);

== matlab function Model_2Systems/Manipulator2 (Tau_fb lose)/Hamiltonian Plant/r-passivity Validation/MATLAB Function ==
  data: Vdot output; q input; qdot input; p input; pdot input; r input; index input; V output; Vr0 parameter
function [Vdot, V] = fcn(q, qdot, p, pdot, r, index, Vr0)

    coder.extrinsic('Manipulator_R');
    V = 0; Vdot = 0;
    [V, Vdot] = Manipulator_R(q, qdot,p, pdot, r, index);
    V = V - Vr0;
end

== matlab function Model_2Systems/Manipulator2 (Tau_fb lose)/Levenberg Compensation ==
  data: q input; tau_k input; z_dot input; tau_c output; index input
function tau_c  = Pre(q, tau_k, z_dot, index)

    coder.extrinsic('Manipulator_Pre');
    tau_c = zeros(2,1);
    [tau_c] = Manipulator_Pre(q, tau_k, z_dot, index);
end

== matlab function Model_2Systems/Manipulator2 (Tau_fb lose)/MATLAB Function1 ==
  data: p input; q input; tau output; tau_dH output; tau_null output; tau_lambda output; tau_fb output; index input
function [tau, tau_dH, tau_null, tau_lambda, tau_fb] = LocalControl(p, q, index)
    

coder.extrinsic('Manipulator_Control');
tau = zeros(3, 1);
tau_dH = zeros(3, 1);
tau_null = zeros(3, 1);
tau_lambda = zeros(3, 1);
tau_fb = zeros(2, 1);
[tau, tau_dH, tau_null, tau_lambda, tau_fb] = Manipulator_Control(q, p, index);

== matlab function Model_2Systems/Manipulator2 (Tau_fb lose)/MATLAB Function2 ==
  data: p input; q input; tau_c input; tau output; tau_fb output; index input
function [tau, tau_fb] = LocalControl(p, q, tau_c, index)
    

coder.extrinsic('Manipulator_OptControl');
tau = zeros(3, 1);
tau_fb = zeros(2, 1);
[tau, tau_fb] = Manipulator_OptControl(q, p, tau_c, index);

== matlab function Model_2Systems/Manipulator/Hamiltonian Plant1/MATLAB Function1 ==
  data: q input; z_out output; p input; r_out output; index input
function [z_out, r_out] = toz(q, p, index)

    coder.extrinsic('Manipulator_z');
    z_out = zeros(2, 1);
    r_out = zeros(2, 1);
    [z_out, r_out] = Manipulator_z(q, p, index);

== matlab function Model_2Systems/Manipulator/Hamiltonian Plant1/MATLAB Function2 ==
  data: q input; qdot output; p input; tau_l input; pdot output; tau_c input; index input
function [qdot, pdot] = fcn(q, p, tau_l, tau_c, index)

    coder.extrinsic('Manipulator_Dynamics');
    qdot = zeros(3, 1);
    pdot = zeros(3, 1);
    [qdot, pdot] = Manipulator_Dynamics(q, p, tau_l, tau_c, index);

== matlab function Model_2Systems/Manipulator2/Hamiltonian Plant1/MATLAB Function1 ==
  data: q input; z_out output; p input; r_out output; index input
function [z_out, r_out] = toz(q, p, index)

    coder.extrinsic('Manipulator_z');
    z_out = zeros(2, 1);
    r_out = zeros(2, 1);
    [z_out, r_out] = Manipulator_z(q, p, index);

== matlab function Model_2Systems/Manipulator2/Hamiltonian Plant1/MATLAB Function2 ==
  data: q input; qdot output; p input; tau_l input; pdot output; tau_c input; index input
function [qdot, pdot] = fcn(q, p, tau_l, tau_c, index)

    coder.extrinsic('Manipulator_Dynamics');
    qdot = zeros(3, 1);
    pdot = zeros(3, 1);
    [qdot, pdot] = Manipulator_Dynamics(q, p, tau_l, tau_c, index);

== matlab function Model_2Systems/Manipulator/MATLAB Function3 ==
  data: p input; q input; tau_c input; tau output; tau_m output; tau_fb output; index input; start_delays parameter
function [tau, tau_m, tau_fb] = LocalControl(p, q, tau_c, index, start_delays)
    

coder.extrinsic('Manipulator_Control');
tau = zeros(3, 1);
tau_fb = zeros(2, 1);
tau_m = zeros(2, 1);
[tau, tau_m, tau_fb] = Manipulator_Control(q, p, tau_c, index, start_delays);

== matlab function Model_2Systems/Manipulator2/MATLAB Function3 ==
  data: p input; q input; tau_c input; tau output; tau_m output; tau_fb output; index input; start_delays parameter
function [tau, tau_m, tau_fb] = LocalControl(p, q, tau_c, index, start_delays)
    

coder.extrinsic('Manipulator_Control');
tau = zeros(3, 1);
tau_fb = zeros(2, 1);
tau_m = zeros(2, 1);
[tau, tau_m, tau_fb] = Manipulator_Control(q, p, tau_c, index, start_delays);

== matlab function Model_2Systems/Edge 1/ST + WVM/WVM ==
  data: t_tilde input; s_in input; r_i input; s_in_prev input; s_out output; tau output; s_hat output; s_buffer output; KL parameter
function [s_out, tau, s_hat, s_buffer]  = fcn(t_tilde, s_in, r_i, s_in_prev, KL)
    s_hat = zeros(2, 1);
    s_buffer = zeros(2, 1);
    s_out = zeros(2, 1);
    tau = zeros(2, 1);
    
    %% If 0 then no new data -> reconstruct!
    % If lower than 0, then the package is reordered and we reject the
    % package
    if(t_tilde <= 0)  
        % WVM
        Y = KL*[s_in_prev; r_i];
        s_hls = Y(3:4);
        
        % If HLS is passive apply HLS
        if(s_hls'*s_hls >= s_in_prev'*s_in_prev)
            s_hat = s_in_prev;
            
        % Otherwise apply the acceptable magnitude in that direction
        else
            s_hat = sign(s_in_prev).*abs(s_hls);
        end

        % Either way repeat the last value
        s_buffer = s_in_prev;
        
    %% If 1 then no weird shenanigans, data arrived on time
    %% If > 1 then the packages are reordered and we keep the last one
    else
        s_hat = s_in; % Use the received value
        s_buffer = s_in; % And store its value
    end    
    Y = KL*[s_hat; r_i];
    tau = Y(1:2); s_out = Y(3:4);

end

== matlab function Model_2Systems/Edge 1/ST + WVM1/WVM ==
  data: t_tilde input; s_in input; r_i input; s_in_prev input; s_out output; tau output; s_hat output; s_buffer output; KR parameter
function [s_out, tau, s_hat, s_buffer]  = fcn(t_tilde, s_in, r_i, s_in_prev, KR)
    s_hat = zeros(2, 1);
    s_buffer = zeros(2, 1);
    s_out = zeros(2, 1);
    tau = zeros(2, 1);
    
    %% If 0 then no new data -> reconstruct!
    % If lower than 0, then the package is reordered and we reject the
    % package
    if(t_tilde <= 0)  
        % WVM
        Y = KR*[s_in_prev; r_i];
        s_hls = Y(3:4);
        
        % If HLS is passive apply HLS
        if(s_hls'*s_hls >= s_in_prev'*s_in_prev)
            s_hat = s_in_prev;
            
        % Otherwise apply the acceptable magnitude in that direction
        else
            s_hat = sign(s_in_prev).*abs(s_hls);
        end

        % Either way repeat the last value
        s_buffer = s_in_prev;
        
    %% If 1 then no weird shenanigans, data arrived on time
    %% If > 1 then the packages are reordered and we keep the last one
    else
        s_hat = s_in; % Use the received value
        s_buffer = s_in; % And store its value
    end    
    Y = KR*[s_hat; r_i];
    tau = Y(1:2); s_out = Y(3:4);

end
